simulink model "HID"  (R2021a)
settings: Solver=VariableStepAuto  StartTime=0.0  StopTime=0.005  MaxStep=1e-4  RelTol=1e-4  EnableMultiTasking=on
libraries: spsSeriesRLCBranchLib x2, spsCurrentMeasurementLib x2, spsVoltageMeasurementLib x2, spsDiodeLib x1, spsMosfetLib x1, spsSeriesRLCLoadLib x1, spsDCVoltageSourceLib x1, spspowerguiLib x1
settings Model: Creator=MathWorks  LastModifiedBy=user
settings SolverCC: AlgebraicLoopSolver=TrustRegion  SolverResetMethod=Robust
settings OptimizationCC: EfficientFloat2IntCast=on  LifeSpan=inf
settings DebuggingCC: ReadBeforeWriteMsg=DisableAll  WriteAfterWriteMsg=DisableAll  WriteAfterReadMsg=DisableAll  UniqueDataStoreMsg=error  StrictBusMsg=ErrorOnBusTreatedAsVector  SFUnexpectedBacktrackingDiag=warning  SFNoUnconditionalDefaultTransitionDiag=warning  SFExecutionAtInitializationDiag=none  SFMachineParentedDataDiag=warning  ArithmeticOperatorsInVariantConditions=warning
settings ModelReferenceCC: UpdateModelReferenceTargets=IfOutOfDate
settings SFSimCC: SFSimEcho=off  SimUseLocalCustomCode=off  CustomCodeUndefinedFunction=UseInterfaceOnly
settings RTWCC: RTWUseLocalCustomCode=off
settings CodeAppCC: StateflowObjectComments=on
settings GRTTargetCC: TargetLangStandard=C89/C90 (ANSI)
settings ConfigComp: CovMetricSettings=dw  CovSaveCumulativeToWorkspaceVar=on  CovSaveSingleToWorkspaceVar=on  CovExternalEMLEnable=off
settings SimscapeCC: SimscapeNormalizeSystem=off  SimscapeNominalValues={1, 'bar'; 1, 'cm^3/s'; 1, 'bar*kg/s'; 1, 'kJ/kg'; 1, 'kW'; }

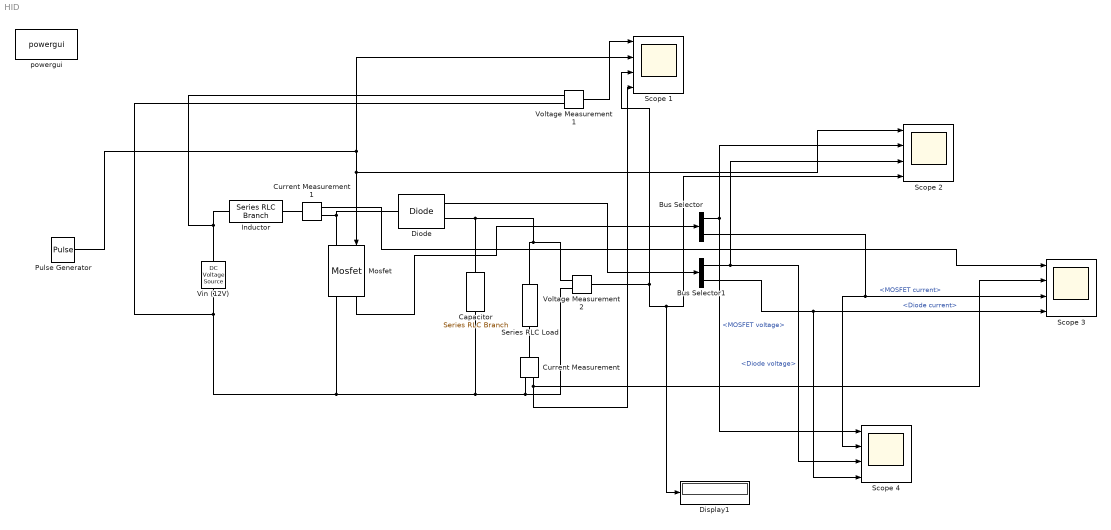
== system HID ==
  Bus Selector : BusSelector  OutputSignals=MOSFET voltage,MOSFET current
  Bus Selector1 : BusSelector  OutputSignals=Diode voltage,Diode current
  Capacitor : spsSeriesRLCBranchLib/Series RLC Branch  LConnTagsString=__new0  RConnTagsString=__new0  BranchType=C  Resistance=1  Inductance=1e-3  SetiL0=off  InitialCurrent=0  Capacitance=2.5e-5  Setx0=off  InitialVoltage=7.5  Measurements=None
  Current Measurement : spsCurrentMeasurementLib/Current Measurement  PhasorSimulation=off  OutputType=Complex  PSBequivalent=0
  Current Measurement1 : spsCurrentMeasurementLib/Current Measurement  PhasorSimulation=off  OutputType=Complex  PSBequivalent=0
  "Diode " : spsDiodeLib/Diode  Ron=0.001  Lon=0  Vf=1.15  IC=0  UseSnubber=0  Rs=500  Cs=250e-9  Measurements=on
  Display1 : Display
  Inductor : spsSeriesRLCBranchLib/Series RLC Branch  LConnTagsString=__new0  RConnTagsString=__new0  BranchType=L  Resistance=1e-3  Inductance=3e-4  SetiL0=off  InitialCurrent=0  Capacitance=1e-6  Setx0=off  InitialVoltage=0  Measurements=None
  "Mosfet " : spsMosfetLib/Mosfet  Ron=0.001  Lon=0  Rd=1e-3  Vfd=0  IC=0  Rs=inf  Cs=inf  Measurements=on
  "Pulse Generator " : DiscretePulseGenerator  PulseType=Time based  Amplitude=5  Period=1/50000  PulseWidth=74
  Scope {1..4} (4 alike) : Scope  NumInputPorts=4
  Series RLC Load : spsSeriesRLCLoadLib/Series RLC Load  LConnTagsString=a  RConnTagsString=__new0  NominalVoltage=12  NominalFrequency=50e3  ActivePower=48  InductivePower=0  CapacitivePower=0  Setx0=off  InitialVoltage=0  SetiL0=off  InitialCurrent=0  Measurements=None  LoadType=constant Z
  Vin (12V) : spsDCVoltageSourceLib/DC Voltage Source  Amplitude=12  Measurements=None
  Voltage Measurement 1 : spsVoltageMeasurementLib/Voltage Measurement  PhasorSimulation=off  OutputType=Complex  PSBequivalent=0
  Voltage Measurement 2 : spsVoltageMeasurementLib/Voltage Measurement  PhasorSimulation=off  OutputType=Complex  PSBequivalent=0
  powergui : spspowerguiLib/powergui  Priority=1  SimulationMode=Continuous  SampleTime=50e-6  frequency=60  Iterations=50  frequencyindice=0  Pbase=100e6  ErrMax=1e-4  UnitsV=kV  UnitsW=MW  buscounter=0  FunctionMessages=off  echomessages=off  EnableUseOfTLC=off  CurrentSourceSwitches=off  DisableSnubberDevices=off  DisableRonSwitches=off  DisableVfSwitches=off  DisplayEquations=off  AutomaticDiscreteSolvers=off  SolverType=Tustin/Backward Euler (TBE)  Interpol=off  ExternalGateDelay=off  methode=off  Ts=100  x0status=blocks  SPID=on  SwTol=0  HookPort=off  NonlinearTolerance=1e-4  nMaxIteration=100  ContinueOnMaxIteration=off  RestoreLinks=warning  ResistiveCurrentMeasurement=off  Frange=[0:2:500]  Ylog=off  Xlog=on  ShowGrid=off  save=off  variable=ZData  structure=0  ZoomFFT=off  StartTime=0.0  cycles=1  DisplayStyle=1  fundamental=60  FreqAxis=off  MaxFrequency=1000  frequencyindicesteady=1  RmsSteady=1  display=off
  wires:
  Voltage Measurement 2/1 -> Scope 1/3, Scope 2/4, Display1/1
  Voltage Measurement 1/1 -> Scope 1/1
  "Pulse Generator "/1 -> Scope 1/2, "Mosfet "/1, Scope 2/1
  "Mosfet "/1 -> Bus Selector/1
  Bus Selector/1 -> Scope 2/2, Scope 4/1  "<MOSFET voltage>"
  "Diode "/1 -> Bus Selector1/1
  Bus Selector1/1 -> Scope 4/3, Scope 2/3  "<Diode voltage>"
  Current Measurement/1 -> Scope 1/4, Scope 3/2
  Bus Selector/2 -> Scope 3/3, Scope 4/2  "<MOSFET current>"
  Bus Selector1/2 -> Scope 4/4, Scope 3/4  "<Diode current>"
  Current Measurement1/1 -> Scope 3/1
  connections:
  "Mosfet "/RConn1 -- Voltage Measurement 1/LConn2 -- Vin (12V)/LConn1 -- Current Measurement/RConn1 -- Voltage Measurement 2/LConn2 -- Capacitor/RConn1
  "Diode "/RConn1 -- Capacitor/LConn1 -- Series RLC Load/LConn1 -- Voltage Measurement 2/LConn1
  Voltage Measurement 1/LConn1 -- Inductor/LConn1 -- Vin (12V)/RConn1
  "Diode "/LConn1 -- Current Measurement1/RConn1 -- "Mosfet "/LConn1
  Current Measurement1/LConn1 -- Inductor/RConn1
  Series RLC Load/RConn1 -- Current Measurement/LConn1
